simulink model "Subsys1_tmp"  (Simulink 8.3)
settings: Solver=FixedStepDiscrete  StartTime=0.0  StopTime=10.0  RelTol=1e-3
settings Model: Creator=sofronis  LastModifiedBy=hbourbou  CovSFcnEnable=on  ExtModeAutoUpdateStatusClock=off
settings DataIOCC: SignalLoggingName=sigsOut
settings DebuggingCC: AlgebraicLoopMsg=error  SaveWithParameterizedLinksMsg=none  SignalResolutionControl=TryResolveAllWithWarning  SolverPrmCheckMsg=none  MultiTaskDSMMsg=warning  MultiTaskCondExecSysMsg=none  FrameProcessingCompatibilityMsg=error  StateNameClashWarn=none
settings HardwareCC: TargetUnknown=on
settings SFSimCC: SimParseCustomCode=off
settings GRTTargetCC: GeneratePreprocessorConditionals=Use local settings

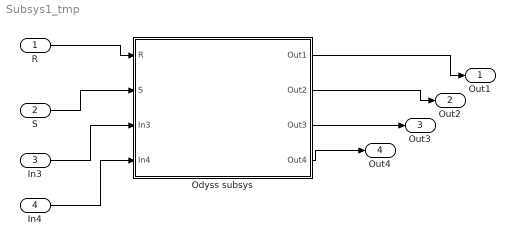
== system Subsys1_tmp ==
  R : Inport  SampleTime=1
  S : Inport  Port=2  SampleTime=1
  In3 : Inport  Port=3  SampleTime=1
  In4 : Inport  Port=4  SampleTime=1
  Odyss subsys : Subsystem
  Out1 : Outport
  Out2 : Outport  Port=2
  Out3 : Outport  Port=3
  Out4 : Outport  Port=4
  wires:
  R/1 -> Odyss subsys/1(R)
  S/1 -> Odyss subsys/2(S)
  In3/1 -> Odyss subsys/3(In3)
  In4/1 -> Odyss subsys/4(In4)
  Odyss subsys/1(Out1) -> Out1/1
  Odyss subsys/2(Out2) -> Out2/1
  Odyss subsys/3(Out3) -> Out3/1
  Odyss subsys/4(Out4) -> Out4/1

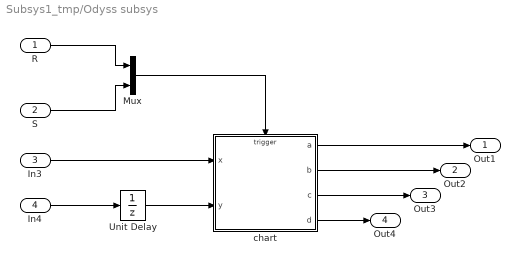
== system Subsys1_tmp/Odyss subsys ==
  R : Inport  SampleTime=1
  S : Inport  Port=2  SampleTime=1
  In3 : Inport  Port=3  SampleTime=1
  In4 : Inport  Port=4  SampleTime=1
  Mux : Mux  Inputs=2
  Unit Delay : UnitDelay  SampleTime=-1
  chart : Stateflow chart  TreatAsAtomicUnit=on
      settings: PermitHierarchicalResolution=ParametersOnly
  Out1 : Outport
  Out2 : Outport  Port=2
  Out3 : Outport  Port=3
  Out4 : Outport  Port=4
  wires:
  R/1 -> Mux/1
  S/1 -> Mux/2
  In3/1 -> chart/1(x)
  Mux/1 -> chart/Trigger
  chart/1(a) -> Out1/1
  chart/2(b) -> Out2/1
  chart/3(c) -> Out3/1
  chart/4(d) -> Out4/1
  In4/1 -> Unit Delay/1
  Unit Delay/1 -> chart/2(y)

== stateflow chart Odyss subsys/chart ==
  state A [parallel]
    settings: executionOrder=1
    state Aa/
      en:a=x+1
    state Ab/
      en:a=x+2
    (default) -> Aa
    Aa -> Ab : S/send(S1,B)
    Ab -> Aa : R/send(R1,B)
  state B [parallel]
    settings: executionOrder=2
    state Ba/
      en:b=x+3
    state Bb/
      en:b=x+4
    (default) -> Ba
    Ba -> Bb : S1/send(S2,C)
    Bb -> Ba : R1/send(R2,C)
  state C [parallel]
    settings: executionOrder=3
    state Ca/
      en:c=x+5
    state Cb/
      en:c=x+6
    (default) -> Ca
    Ca -> Cb : S2/send(S3,D)
    Cb -> Ca : R2/send(R3,D)
  state D [parallel]
    settings: executionOrder=4
    state Da/
      en:d=x+7
    state Db/
      en:d=x+8
    (default) -> Da
    Da -> Db : S3
    Db -> Da : R3
  data: a output int32; x input int32; b output int32; c output int32; d output int32; y input int32
  events: R1 local EITHER_EDGE_EVENT; S1 local EITHER_EDGE_EVENT; R input RISING_EDGE_EVENT; S input FALLING_EDGE_EVENT; R2 local EITHER_EDGE_EVENT; S2 local EITHER_EDGE_EVENT; S3 local EITHER_EDGE_EVENT; R3 local EITHER_EDGE_EVENT
